simulink model "Arm_Control_Tuning_v002"  (R2017b)
settings: Solver=FixedStepAuto  StartTime=0.0  StopTime=30.0  FixedStep=0.02  MaxStep=0.01  RelTol=1e-3
InitFcn:
  | deg=pi/180;
libraries: simulink x1
settings Model: Creator=Martin  LastModifiedBy=GEH-Magnet School 1

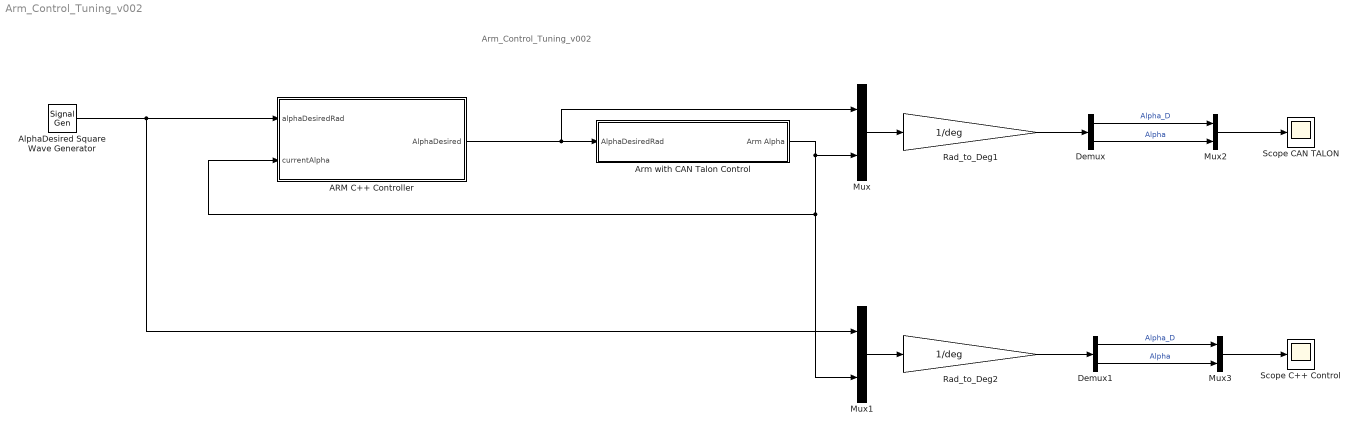
== system Arm_Control_Tuning_v002 ==
  note: Arm_Control_Tuning_v002
  ARM C++ Controller : Subsystem
  AlphaDesired Square Wave Generator : SignalGenerator  WaveForm=square  Amplitude=90*deg  Frequency=0.1
  "Arm with CAN Talon Control " : Subsystem
  Demux : Demux  Outputs=2
  Demux1 : Demux  Outputs=2
  Mux{,1..3} (4 alike) : Mux  Inputs=2
  Rad_to_Deg1 : Gain  Gain=1/deg
  Rad_to_Deg2 : Gain  Gain=1/deg
  Scope C++ Control : Scope
  Scope CAN TALON : Scope
  wires:
  ARM C++ Controller/1(AlphaDesired) -> Mux/1, "Arm with CAN Talon Control "/1(AlphaDesiredRad)
  Mux/1 -> Rad_to_Deg1/1
  "Arm with CAN Talon Control "/1(Arm Alpha) -> Mux1/2, ARM C++ Controller/2(currentAlpha), Mux/2
  AlphaDesired Square Wave Generator/1 -> Mux1/1, ARM C++ Controller/1(alphaDesiredRad)
  Mux1/1 -> Rad_to_Deg2/1
  Rad_to_Deg1/1 -> Demux/1
  Demux/1 -> Mux2/1  "Alpha_D"
  Mux2/1 -> Scope CAN TALON/1
  Demux/2 -> Mux2/2  "Alpha"
  Demux1/2 -> Mux3/2  "Alpha"
  Mux3/1 -> Scope C++ Control/1
  Demux1/1 -> Mux3/1  "Alpha_D"
  Rad_to_Deg2/1 -> Demux1/1

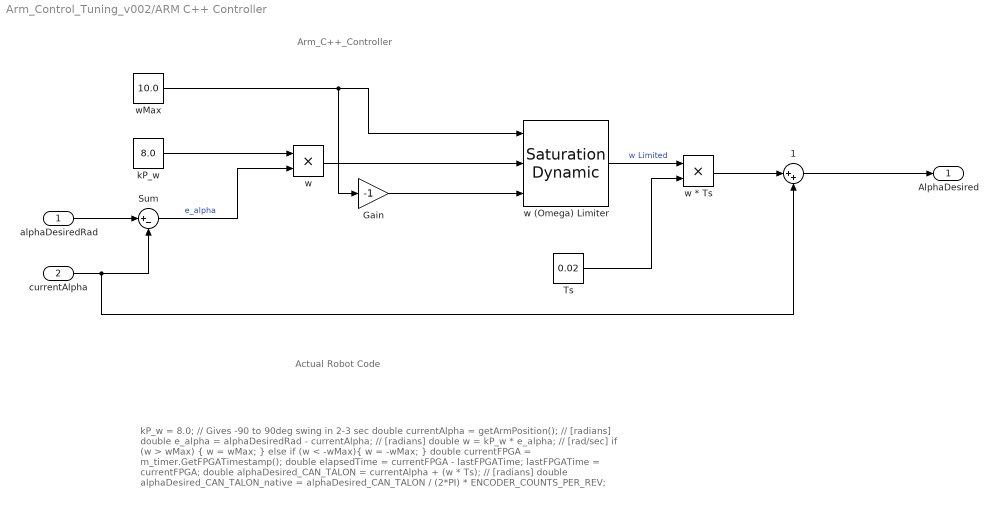
== system Arm_Control_Tuning_v002/ARM C++ Controller ==
  note: kP_w = 8.0;		// Gives -90 to 90deg swing in 2-3 sec
      |
      | double currentAlpha = getArmPosition();						// [radians]
      | double e_alpha = alphaDesiredRad - currentAlpha; 			// [radians]
      | double w = kP_w * e_alpha;									// [rad/sec]
      | if (w > wMax) {		w = wMax;	}	else if (w < -wMax){		w = -wMax;	}
      |
      | double currentFPGA = m_timer.GetFPGATimestamp();
      | double elapsedTime = currentFPGA - lastFPGATime;
      | 	lastFPGATime = currentFPGA;
      | double alphaDesired_CAN_TALON = currentAlpha + (w * Ts);		// [radians]
      | double alphaDesired_CAN_TALON_native = alphaDesired_CAN_TALON / (2*PI) * ENCODER_COUNTS_PER_REV;
  note: Arm_C++_Controller
  note: Actual Robot Code
  alphaDesiredRad : Inport
  currentAlpha : Inport  Port=2
  1 : Sum  Inputs=|++
  Gain : Gain  Gain=-1
  Sum : Sum  Inputs=|+-
  Ts : Constant  Value=0.02
  "kP_w " : Constant  Value=8.0
  w : Product
  w (Omega) Limiter : simulink/Discontinuities/Saturation Dynamic  OutMin=[]  OutMax=[]  OutDataTypeStr=Inherit: Same as second input  OutDataType=fixdt(1, 16)  OutScaling=2^-10  DoSatur=off
  w * Ts : Product
  "wMax " : Constant  Value=10.0
  AlphaDesired : Outport
  wires:
  alphaDesiredRad/1 -> Sum/1
  currentAlpha/1 -> Sum/2, 1/2
  Sum/1 -> w/2  "e_alpha"
  "kP_w "/1 -> w/1
  w/1 -> w (Omega) Limiter/2
  "wMax "/1 -> Gain/1, w (Omega) Limiter/1
  w (Omega) Limiter/1 -> w * Ts/1  "w Limited"
  Ts/1 -> w * Ts/2
  w * Ts/1 -> 1/1
  Gain/1 -> w (Omega) Limiter/3
  1/1 -> AlphaDesired/1

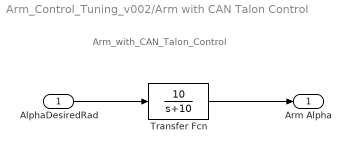
== system Arm_Control_Tuning_v002/Arm with CAN Talon Control  ==
  note: Arm_with_CAN_Talon_Control
  AlphaDesiredRad : Inport
  Transfer Fcn : TransferFcn  Numerator=10  Denominator=[1 10]
  Arm Alpha : Outport
  wires:
  AlphaDesiredRad/1 -> Transfer Fcn/1
  Transfer Fcn/1 -> Arm Alpha/1
